simulink model "DeltaSigma_ADC"  (R2026a)
settings: Solver=FixedStepAuto  FixedStep=1/F_s
values from neighbouring files (symbols this model uses):
  A_in = 0.3    [Matlab.mat]
undefined symbols (not defined in the file or in its folder): DC_in, DiscIntNeverNeededParam, F_in, F_s, OSR
libraries: dspmlti4 x1
settings Model: Creator=KMStudios  LastModifiedBy=KMStudios

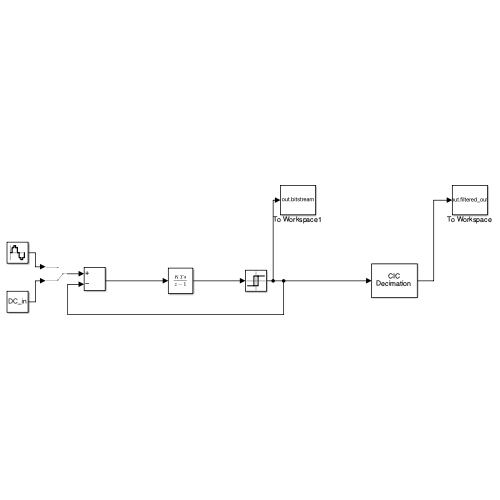
[thumbnail: Simulink's stored preview of the top-level diagram]
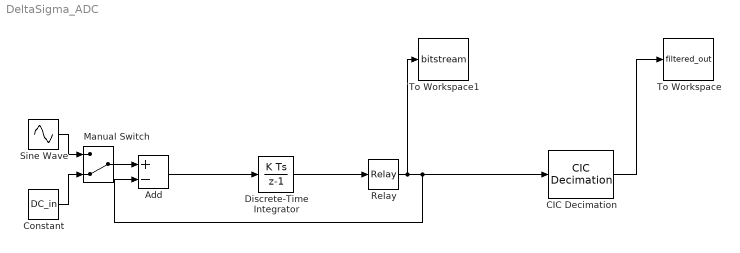
== system DeltaSigma_ADC ==
  Add : Sum  Inputs=+-  OutDataTypeStr=double  AccumDataTypeStr=double
  CIC Decimation : dspmlti4/CIC Decimation  filtFrom=Dialog parameters  filtobj=CICDECIM  ftype=Decimator  R=OSR  M=1  N=3  filterInternals=Full precision  BPS=[16 16 16 16]  FLPS=0  outputWordLength=32  outputFracLength=0  launchFVT=off  framing=Maintain input frame rate  RateOptions=Allow multirate processing
  Constant : Constant  Value=DC_in
  Discrete-Time Integrator : DiscreteIntegrator  SampleTime=1/F_s  OutDataTypeStr=double  ICPrevOutput=DiscIntNeverNeededParam  ICPrevScaledInput=DiscIntNeverNeededParam
  Manual Switch : ManualSwitch  CurrentSetting=0
  Relay : Relay  OnSwitchValue=0  OffSwitchValue=0  OffOutputValue=-1  OutDataTypeStr=int64
  Sine Wave : Sin  Amplitude=A_in  Frequency=2*pi*F_in  SampleTime=1/F_s
  To Workspace : ToWorkspace  VariableName=filtered_out  SampleTime=-1
      settings: Save2DSignal=2-D array (concatenate along first dimension)
  To Workspace1 : ToWorkspace  VariableName=bitstream  SampleTime=-1
      settings: Save2DSignal=2-D array (concatenate along first dimension)
  wires:
  Add/1 -> Discrete-Time Integrator/1
  Discrete-Time Integrator/1 -> Relay/1
  CIC Decimation/1 -> To Workspace/1
  Relay/1 -> To Workspace1/1, CIC Decimation/1, Add/2
  Sine Wave/1 -> Manual Switch/1
  Manual Switch/1 -> Add/1
  Constant/1 -> Manual Switch/2
